simulink model "pneumatiques"  (R2024b)
settings: Solver=FixedStepAuto  StartTime=0.0  StopTime=1  FixedStep=Ts  RelTol=1e-3
settings Model: Creator=marti  LastModifiedBy=marti

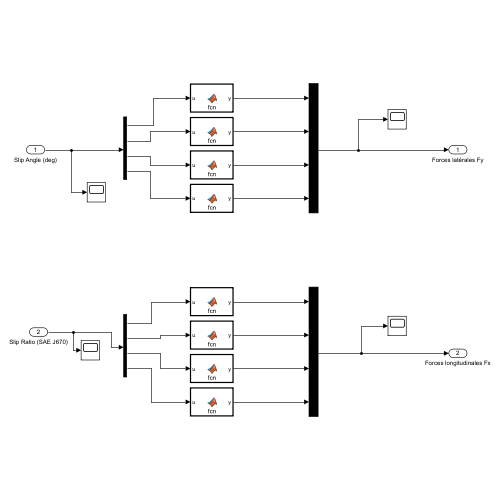
[thumbnail: Simulink's stored preview of the top-level diagram]
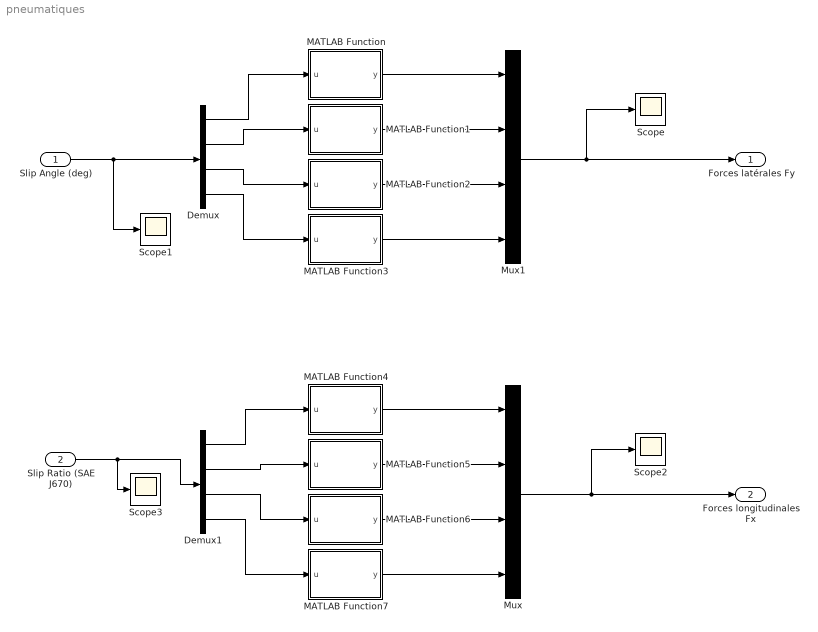
== system pneumatiques ==
  Slip Angle (deg) : Inport
  Slip Ratio (SAE J670) : Inport  Port=2
  Demux : Demux
  Demux1 : Demux
  MATLAB Function : MATLAB Function  TreatAsAtomicUnit=on
  MATLAB Function1 : MATLAB Function  TreatAsAtomicUnit=on
  MATLAB Function2 : MATLAB Function  TreatAsAtomicUnit=on
  MATLAB Function3 : MATLAB Function  TreatAsAtomicUnit=on
  MATLAB Function4 : MATLAB Function  TreatAsAtomicUnit=on
  MATLAB Function5 : MATLAB Function  TreatAsAtomicUnit=on
  MATLAB Function6 : MATLAB Function  TreatAsAtomicUnit=on
  MATLAB Function7 : MATLAB Function  TreatAsAtomicUnit=on
  Mux : Mux
  Mux1 : Mux
  Scope{,1..3} (4 alike) : Scope
  Forces latérales Fy : Outport
  Forces longitudinales Fx : Outport  Port=2
  wires:
  Slip Angle (deg)/1 -> Scope1/1, Demux/1
  Slip Ratio (SAE J670)/1 -> Scope3/1, Demux1/1
  Demux/3 -> MATLAB Function2/1(u)
  Demux/2 -> MATLAB Function1/1(u)
  Demux/1 -> MATLAB Function/1(u)
  Demux/4 -> MATLAB Function3/1(u)
  Demux1/3 -> MATLAB Function6/1(u)
  Demux1/2 -> MATLAB Function5/1(u)
  Demux1/1 -> MATLAB Function4/1(u)
  Demux1/4 -> MATLAB Function7/1(u)
  MATLAB Function4/1(y) -> Mux/1
  MATLAB Function5/1(y) -> Mux/2
  MATLAB Function6/1(y) -> Mux/3
  MATLAB Function7/1(y) -> Mux/4
  MATLAB Function/1(y) -> Mux1/1
  MATLAB Function1/1(y) -> Mux1/2
  MATLAB Function2/1(y) -> Mux1/3
  MATLAB Function3/1(y) -> Mux1/4
  Mux1/1 -> Scope/1, Forces latérales Fy/1
  Mux/1 -> Scope2/1, Forces longitudinales Fx/1

== matlab function pneumatiques/MATLAB Function ==
  data: u input; y output
function y = fcn(u)
    B=10.48;
    C=-1.75;
    D=1784.7;
    E=0.44;
    y = D*sin(C*atan(B*u-E*(B*u-atan(B*u))));
end

== matlab function pneumatiques/MATLAB Function2 ==
  data: u input; y output
function y = fcn(u)
    B=10.48;
    C=-1.75;
    D=1784.7;
    E=0.44;
    y = D*sin(C*atan(B*u-E*(B*u-atan(B*u))));
end

== matlab function pneumatiques/MATLAB Function3 ==
  data: u input; y output
function y = fcn(u)
    u_rad=pi/180*u;
    B=10.48;
    C=-1.75;
    D=1784.7;
    E=0.44;
    y = D*sin(C*atan(B*u_rad-E*(B*u_rad-atan(B*u_rad))));
end

== matlab function pneumatiques/MATLAB Function4 ==
  data: u input; y output
function y = fcn(u)
    B=12;
    C=1.55;
    D=1500;
    E=-1;
    y = D*sin(C*atan(B*u-E*(B*u-atan(B*u))));
end

== matlab function pneumatiques/MATLAB Function5 ==
  data: u input; y output
function y = fcn(u)
    B=12;
    C=1.55;
    D=1500;
    E=-1;
    y = D*sin(C*atan(B*u-E*(B*u-atan(B*u))));
end

== matlab function pneumatiques/MATLAB Function6 ==
  data: u input; y output
function y = fcn(u)
    B=12;
    C=1.55;
    D=1500;
    E=-1;
    y = D*sin(C*atan(B*u-E*(B*u-atan(B*u))));
end

== matlab function pneumatiques/MATLAB Function7 ==
  data: u input; y output
function y = fcn(u)
    B=12;
    C=1.55;
    D=1500;
    E=-1;
    y = D*sin(C*atan(B*u-E*(B*u-atan(B*u))));
end

== matlab function pneumatiques/MATLAB Function1 ==
  data: u input; y output
function y = fcn(u)
    B=10.48;
    C=-1.75;
    D=1784.7;
    E=0.44;
    y = D*sin(C*atan(B*u-E*(B*u-atan(B*u))));
end
